simulink model "auditory_nerve"  (R2020b)
settings: Solver=FixedStepDiscrete  StartTime=0.0  StopTime=stopTime  FixedStep=2.0833333333333333e-05  RelTol=1e-3
values from neighbouring files (symbols this model uses):
  delay_point = max(0,ceil(delay/tdres))    [modelparameters.m]
settings Model: Creator=Ross  LastModifiedBy=dack
settings DataIOCC: SaveOutput=off  SaveTime=off  ReturnWorkspaceOutputs=off
settings OptimizationCC: BlockReduction=off  ConditionallyExecuteInputs=off  DefaultParameterBehavior=Inlined
settings DebuggingCC: ReadBeforeWriteMsg=DisableAll  WriteAfterWriteMsg=DisableAll  WriteAfterReadMsg=DisableAll  AlgebraicLoopMsg=error  MultiTaskDSMMsg=none  SingleTaskRateTransMsg=error  PregeneratedLibrarySubsystemCodeDiagnostic=none  ArithmeticOperatorsInVariantConditions=warning
settings HardwareCC: ProdBitPerPointer=32  ProdBitPerSizeT=32  ProdBitPerPtrDiffT=32  ProdLargestAtomicFloat=None  ProdIntDivRoundTo=Undefined  ProdEndianess=Unspecified  ProdWordSize=32  ProdHWDeviceType=ASIC/FPGA->ASIC/FPGA  TargetBitPerPointer=64  TargetBitPerSizeT=64  TargetBitPerPtrDiffT=64  TargetLongLongMode=on  TargetIntDivRoundTo=Zero  TargetEndianess=LittleEndian  TargetWordSize=64  TargetHWDeviceType=Custom Processor->MATLAB Host Computer  ProdEqTarget=off
settings ModelReferenceCC: UpdateModelReferenceTargets=IfOutOfDate  ModelReferenceNumInstancesAllowed=Single
settings SFSimCC: SFSimEcho=off  SimUseLocalCustomCode=off  CustomCodeUndefinedFunction=UseInterfaceOnly
settings RTWCC: RTWUseLocalCustomCode=off

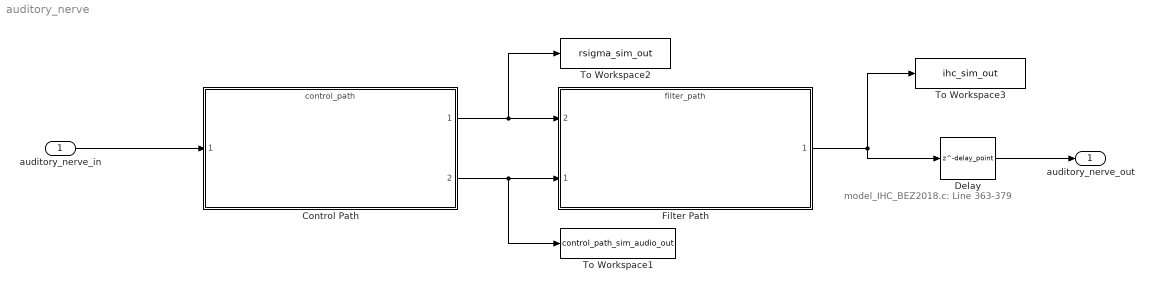
== system auditory_nerve ==
  note: model_IHC_BEZ2018.c: Line 363-379
  auditory_nerve_in : Inport  OutDataTypeStr=single  PortDimensions=1  SampleTime=[2.0833333333333333e-05,0]
  Control Path : ModelReference  ModelNameDialog=control_path.slx  SimulationMode=Normal  ModelReferenceVersion=1.167
  Delay : Delay  DelayLength=delay_point
  Filter Path : ModelReference  ModelNameDialog=filter_path.slx  SimulationMode=Normal  ModelReferenceVersion=1.136
      settings: PortSchema="{\"entries\":[{\"content\":{\"sides\":[{\"content\":{\"connectorIds\":[\"In2\",\"In1\"]},\"type\":\"ConnectorPlacement.EquallySpacedRectSide\",\"uuid\":\"a938cdcf-4bcd-4410-817f-50684eac1b21\"},{\"content\":{\"connectorIds\":[\"Out1\"],\"side\":\"RIGHT\"},\"type\":\"ConnectorPlacement.EquallySpacedRectSide\",\"uuid\":\"ab44b41a-26af-4f52-8ccb-573e2672bd4c\"},{\"content\":{\"connectorIds\":[],\"side\":\"TOP\"},\"type\":\"ConnectorPlacement.EquallySpacedRectSide\",\"uuid\":\"130442d1-41b4-41cf-b390-fc44af304efe\"},{\"content\":{\"connectorIds\":[],\"side\":\"HIDDEN\"},\"type\":\"ConnectorPlacement.EquallySpacedRectSide\",\"uuid\":\"0566c7e3-1e0f-4faa-8bf9-1c8c3f1e33bc\"}]},\"type\":\"ConnectorPlacement.EquallySpacedConnector\",\"uuid\":\"14674991-f311-4310-8a62-4bd572ddd374\"}],\"packageUris\":[\"http://schema.mathworks.com/mf0/Connector/R2020b\"],\"version\":\"1.0\"}"
  To Workspace1 : ToWorkspace  VariableName=control_path_sim_audio_out  SampleTime=-1
  To Workspace2 : ToWorkspace  VariableName=rsigma_sim_out  SampleTime=-1
  To Workspace3 : ToWorkspace  VariableName=ihc_sim_out  SampleTime=-1
  auditory_nerve_out : Outport
  wires:
  auditory_nerve_in/1 -> Control Path/1
  Control Path/1 -> Filter Path/2, To Workspace2/1
  Control Path/2 -> To Workspace1/1, Filter Path/1
  Filter Path/1 -> Delay/1, To Workspace3/1
  Delay/1 -> auditory_nerve_out/1
